simulink library "main_rotor"  (R2022b)
settings: Solver=VariableStepAuto  StartTime=0.0  StopTime=10.0  RelTol=1e-3
undefined symbols (not defined in the file or in its folder): plant_sample_time_s, universal_constants, veh_params
libraries: flapping_dynamics x1, mr_thrust x1
settings Model: Creator=Tanmay.Mandal  LastModifiedBy=Tanmay.Mandal

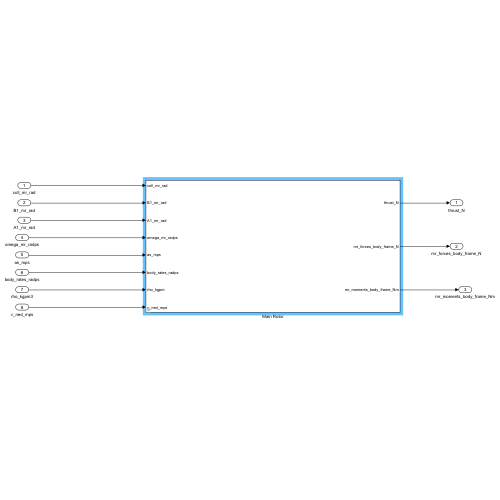
[thumbnail: Simulink's stored preview of the top-level diagram]
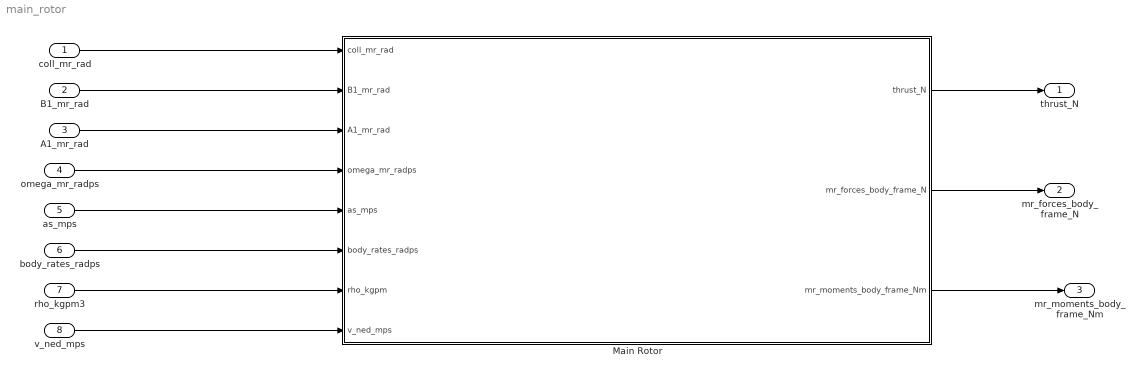
== system main_rotor ==
  coll_mr_rad : Inport
  B1_mr_rad : Inport  Port=2
  A1_mr_rad : Inport  Port=3
  omega_mr_radps : Inport  Port=4
  as_mps : Inport  Port=5
  body_rates_radps : Inport  Port=6
  rho_kgpm3 : Inport  Port=7
  v_ned_mps : Inport  Port=8  OutDataTypeStr=double  Unit=m/s  PortDimensions=[3, 1]
  Main Rotor : Subsystem  mask{veh_params=veh_params, universal_constants=universal_constants}
      mask prompts: veh_params "Vehicle Parameters Struct"; universal_constants "Universal Parameters Struct"
  thrust_N : Outport
  mr_forces_body_frame_N : Outport  Port=2  OutDataTypeStr=double  Unit=N  PortDimensions=[3, 1]
  mr_moments_body_frame_Nm : Outport  Port=3  OutDataTypeStr=double  Unit=N*m  PortDimensions=[3, 1]
  wires:
  coll_mr_rad/1 -> Main Rotor/1(coll_mr_rad)
  B1_mr_rad/1 -> Main Rotor/2(B1_mr_rad)
  A1_mr_rad/1 -> Main Rotor/3(A1_mr_rad)
  omega_mr_radps/1 -> Main Rotor/4(omega_mr_radps)
  as_mps/1 -> Main Rotor/5(as_mps)
  body_rates_radps/1 -> Main Rotor/6(body_rates_radps)
  rho_kgpm3/1 -> Main Rotor/7(rho_kgpm)
  v_ned_mps/1 -> Main Rotor/8(v_ned_mps)
  Main Rotor/1(thrust_N) -> thrust_N/1
  Main Rotor/2(mr_forces_body_frame_N) -> mr_forces_body_frame_N/1
  Main Rotor/3(mr_moments_body_frame_Nm) -> mr_moments_body_frame_Nm/1

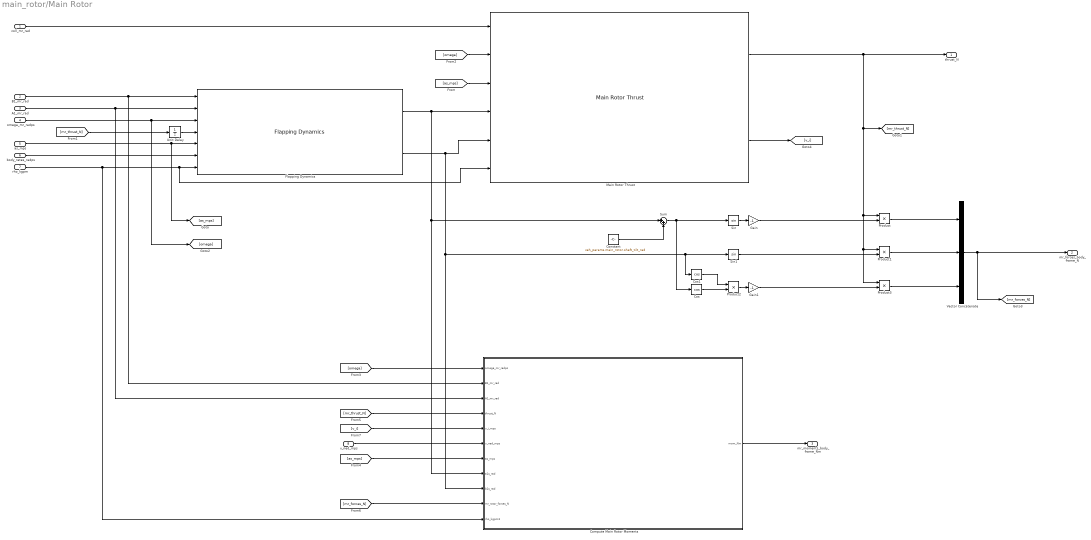
== system main_rotor/Main Rotor ==
  coll_mr_rad : Inport
  B1_mr_rad : Inport  Port=2
  A1_mr_rad : Inport  Port=3
  omega_mr_radps : Inport  Port=4
  as_mps : Inport  Port=5
  body_rates_radps : Inport  Port=6
  rho_kgpm : Inport  Port=7
  v_ned_mps : Inport  Port=8  OutDataTypeStr=double  Unit=m/s  PortDimensions=[3, 1]
  Compute Main Rotor Moments : MATLAB Function  TreatAsAtomicUnit=on  mask{veh_params=veh_params, universal_constants=universal_constants}
      mask prompts: veh_params "Vehicle Parameters Struct"; universal_constants "Universal Constants Struct"
  Constant : Constant  Value=veh_params.main_rotor.shaft_tilt_rad  SampleTime=plant_sample_time_s
  Cos : Trigonometry  Operator=cos
  Cos1 : Trigonometry  Operator=cos
  Flapping Dynamics : flapping_dynamics/Flapping Dynamics  SystemSampleTime=-1  VariantActivationTime=update diagram  Latency=0  AutoFrameSizeCalculation=off
  Gain : Gain  Gain=-1
  Gain1 : Gain  Gain=-1
  Main Rotor Thrust : mr_thrust/Main Rotor Thrust  SystemSampleTime=-1  VariantActivationTime=update diagram  Latency=0  AutoFrameSizeCalculation=off
  Product{,1..3} (4 alike) : Product
  Sin : Trigonometry
  Sin1 : Trigonometry
  Sum : Sum  Inputs=|++
  Unit Delay : UnitDelay  SampleTime=-1  HasFrameUpgradeWarning=on
  Vector Concatenate : Concatenate  NumInputs=3
  thrust_N : Outport
  mr_forces_body_frame_N : Outport  Port=2  OutDataTypeStr=double  Unit=N  PortDimensions=[3, 1]
  mr_moments_body_frame_Nm : Outport  Port=3  OutDataTypeStr=double  Unit=N*m  PortDimensions=[3, 1]
  wires:
  as_mps/1 -> [as_mps], Flapping Dynamics/5
  [mr_thrust_N] -> Unit Delay/1
  Product1/1 -> Vector Concatenate/2
  [as_mps] -> Main Rotor Thrust/3
  [omega] -> Main Rotor Thrust/2
  [mr_thrust_N] -> Compute Main Rotor Moments/4(thrust_N)
  [v_i] -> Compute Main Rotor Moments/5(v_i_mps)
  [as_mps] -> Compute Main Rotor Moments/7(as_mps)
  Main Rotor Thrust/2 -> [v_i]
  Gain1/1 -> Product3/2
  rho_kgpm/1 -> Compute Main Rotor Moments/11(rho_kgpm3), Main Rotor Thrust/6, Flapping Dynamics/7
  Sum/1 -> Sin/1, Cos/1
  Product/1 -> Vector Concatenate/1
  [omega] -> Compute Main Rotor Moments/1(omega_mr_radps)
  Product3/1 -> Vector Concatenate/3
  Flapping Dynamics/2 -> Compute Main Rotor Moments/9(b1s_rad), Cos1/1, Sin1/1, Main Rotor Thrust/5
  A1_mr_rad/1 -> Compute Main Rotor Moments/3(A1_mr_rad), Flapping Dynamics/2
  Flapping Dynamics/1 -> Compute Main Rotor Moments/8(a1s_rad), Sum/1, Main Rotor Thrust/4
  omega_mr_radps/1 -> [omega], Flapping Dynamics/3
  B1_mr_rad/1 -> Compute Main Rotor Moments/2(B1_mr_rad), Flapping Dynamics/1
  Product2/1 -> Gain1/1
  Constant/1 -> Sum/2
  Sin/1 -> Gain/1
  Sin1/1 -> Product1/2
  Unit Delay/1 -> Flapping Dynamics/4
  Cos1/1 -> Product2/1
  Cos/1 -> Product2/2
  [mr_forces_N] -> Compute Main Rotor Moments/10(mr_rotor_forces_N)
  Gain/1 -> Product/2
  v_ned_mps/1 -> Compute Main Rotor Moments/6(v_ned_mps)
  coll_mr_rad/1 -> Main Rotor Thrust/1
  body_rates_radps/1 -> Flapping Dynamics/6
  Main Rotor Thrust/1 -> thrust_N/1, Product/1, Product1/1, Product3/1, [mr_thrust_N]
  Compute Main Rotor Moments/1(mom_Nm) -> mr_moments_body_frame_Nm/1
  Vector Concatenate/1 -> mr_forces_body_frame_N/1, [mr_forces_N]

== matlab function main_rotor/Main Rotor/Compute Main Rotor Moments ==
  data: omega_mr_radps input double size=1; mom_Nm output double size=[3, 1]; B1_mr_rad input double size=1; A1_mr_rad input double size=1; thrust_N input double size=1; v_i_mps input double size=1; v_ned_mps input double size=[3, 1]; as_mps input double size=[3, 1]; a1s_rad input double size=1; b1s_rad input double size=1; mr_rotor_forces_N input double size=[3, 1]; rho_kgpm3 input double size=1; veh_params parameter; universal_constants parameter
function mom_Nm = main_rotor_moments(omega_mr_radps, B1_mr_rad, A1_mr_rad, thrust_N, v_i_mps, ...
                                     v_ned_mps, as_mps, a1s_rad, b1s_rad, ...
                                     mr_rotor_forces_N, rho_kgpm3, veh_params, universal_constants)
%MAIN_ROTOR_MOMENTS Computes moments in body axis generated by the
%main rotor
%
%Inputs:
%omega_mr_radps                 : Main rotor angular velocity
%B1_mr_rad                      : Cyclic pitch input
%A1_mr_rad                      : Cyclic roll input
%thrust_N                       : Main rotor thrust
%v_i_mps                        : Induced velocity at main rotor
%v_ned_mps                      : NED velocity
%as_mps                         : Airspeed vector in body axis
%a1s_rad                        : Longitudinal flap angle 
%b1s_rad                        : Lateral flap angle
%main_rotor_forces_N            : Forces due to main rotor in body axis
%rho_kgpm3                      : Altitude corrected air density
%veh_params                         : Vehicle parameters struct
%universal_constants            : Structure with universal constants
%
%Outputs:
%mom_Nm                         : Moments in body axis due to main rotor

mom_Nm = main_rotor_moments_function(omega_mr_radps, B1_mr_rad, A1_mr_rad, thrust_N, v_i_mps, ...
                                     v_ned_mps, as_mps, a1s_rad, b1s_rad, ...
                                     mr_rotor_forces_N, rho_kgpm3, veh_params, universal_constants);

end
